simulink model "H2DFRL_LExCI_env"  (R2023a)
settings: Solver=FixedStepAuto  StartTime=0.0  StopTime=50  FixedStep=0.08  RelTol=1e-3
values from neighbouring files (symbols this model uses):
  action_mean_selector_ppo = 1:num_actions    [ReinforcementLearningBlockInit_H2DFRL.m]
  action_sampling_mode = 1    [ReinforcementLearningBlockInit_H2DFRL.m]
  action_selector_ddpg = 1:num_actions    [ReinforcementLearningBlockInit_H2DFRL.m]
  action_std_selector_ppo = 1:num_actions    [ReinforcementLearningBlockInit_H2DFRL.m]
  action_type = 1    [ReinforcementLearningBlockInit_H2DFRL.m]
  C2C_NMPC = init_C2C_NMPC_H2DF(C2C_NMPC.expdata)    [init_H2DFRL_GRU.m]
  LowerLimit = ([0.17e-3;350;-5;1e-3] - C2C_NMPC.Normalization.controls.mean)./(C2C_NMPC.Normalization.controls.std)    [init_H2DFRL_GRU.m]
  num_actions = 4    [ReinforcementLearningBlockInit_H2DFRL.m]
  rl_algorithm = 1    [ReinforcementLearningBlockInit_H2DFRL.m]
  UpperLimit = ([0.5e-3;900;2;5.5e-3] - C2C_NMPC.Normalization.controls.mean)./(C2C_NMPC.Normalization.controls.std)    [init_H2DFRL_GRU.m]
undefined symbols (not defined in the file or in its folder): CA50_offset, DiscIntNeverNeededParam, enable_CA50_noise, enable_CA50_offset, enable_IMEP_noise, enable_IMEP_offset, IMEP_offset, NUMBER_OF_ACTIONS
libraries: simulink x15, dspsrcs4 x4
(part 2 of 4)

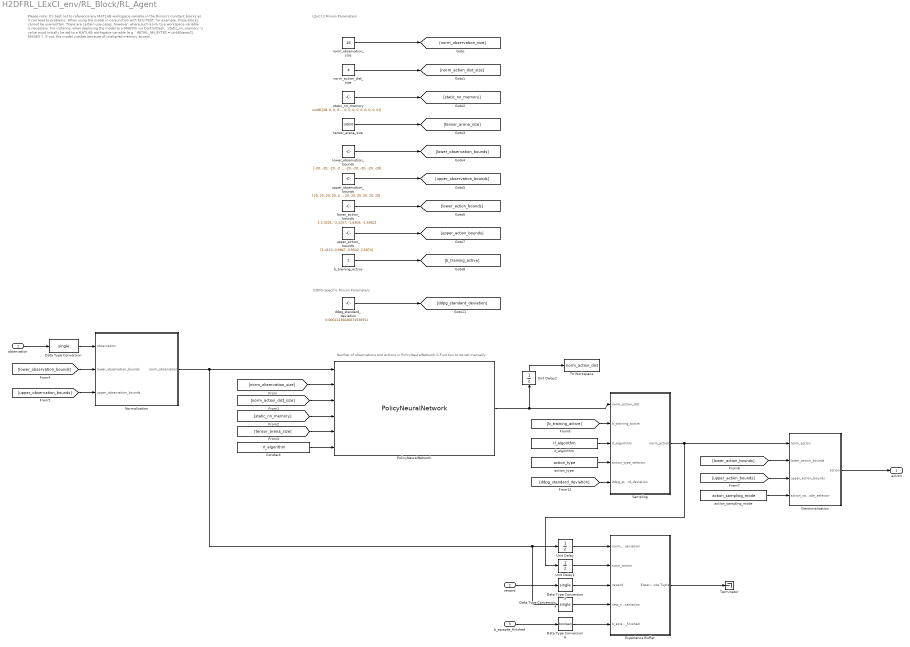
== system H2DFRL_LExCI_env/RL_Block/RL_Agent ==
  note: LExCI 2 Minion Parameters
  note: DDPG-Specific Minion Parameters
  note: Number of observations and actions in PolicyNeuralNetwork S-Function to be set manually.
  note: Please note:
      |
      | It's best not to reference any MATLAB workspace variable in the Minion's constant blocks as it can lead to
      | problems. When using the model in conjunction with ECU-TEST, for example, those blocks cannot be
      | overwritten.
      |
      | There are certain use-cases, however, where such a link to a workspace variable is necessary. For
      | instance, when deploying the model to a MABXIII via ControlDesk, `static_nn_memory`'s value must
      | initially be set to a MATLAB workspace variable (e.g. `INITIAL_NN_BYTES = uint8(zeros(1, 65536))`). If
      | not, the model crashes because of unaligned memory access.
  observation : Inport
  reward : Inport  Port=2
  b_episode_finished : Inport  Port=3
  Constant : Constant  Value=rl_algorithm  OutDataTypeStr=uint32
  Data Type Conversion : DataTypeConversion  OutDataTypeStr=single  SaturateOnIntegerOverflow=off  RndMeth=Floor
  Data Type Conversion3 : DataTypeConversion  OutDataTypeStr=single  SaturateOnIntegerOverflow=off  RndMeth=Floor
  Data Type Conversion4 : DataTypeConversion  OutDataTypeStr=single  SaturateOnIntegerOverflow=off  RndMeth=Floor
  Data Type Conversion6 : DataTypeConversion  OutDataTypeStr=boolean  SaturateOnIntegerOverflow=off  RndMeth=Floor
  Denormalization : Subsystem
  Experience Buffer : Subsystem
  Normalization : Subsystem
  PolicyNeuralNetwork : S-Function  InitFcn=try, set_param(gcb,'FunctionName','PolicyNeuralNetwork'), end  FunctionName=PolicyNeuralNetwork  SFunctionModules=PolicyNeuralNetwork_wrapper.cpp activations activations_common add add_common add_n arg_min_max assign_variable batch_to_space_nd broadcast_args broadcast_to call_once cast ceil circular_buffer circular_buffer_common comparisons concatenation conv conv_common cumsum depth_to_space depthwise_conv depthwise_conv_common dequantize dequantize_common detection_postprocess div elementwise elu ethosu exp expand_dims fill floor floor_div floor_mod fully_connected fully_connected_common gather gather_nd hard_swish hard_swish_common if kernel_runner kernel_util_micro l2norm l2_pool_2d leaky_relu leaky_relu_common logical logical_common logistic logistic_common log_softmax lstm_eval maximum_minimum micro_tensor_utils mirror_pad mul mul_common neg pack pad pooling pooling_common prelu prelu_common quantize quantize_common read_variable reduce reduce_common reshape resize_bilinear resize_nearest_neighbor round shape slice softmax softmax_common space_to_batch_nd space_to_depth split split_v squared_difference squeeze strided_slice sub sub_common svdf svdf_common tanh transpose transpose_conv unidirectional_sequence_lstm unpack var_handle while zeros_like flatbuffer_conversions op_resolver tensor_utils error_reporter schema_utils kernel_util portable_tensor_utils quantization_util common memory_helpers all_ops_resolver micro_graph micro_error_reporter micro_context micro_profiler test_helpers recording_micro_allocator micro_interpreter micro_time micro_resource_variable test_helper_custom_ops flatbuffer_utils mock_micro_graph debug_log micro_allocation_info system_setup micro_allocator micro_string micro_utils fake_micro_context persistent_arena_buffer_allocator recording_single_arena_buffer_allocator non_persistent_arena_buffer_allocator single_arena_buffer_allocator greedy_memory_planner linear_memory_planner non_persistent_buffer_planner_shim  SFunctionDeploymentMode=off  EnableBusSupport=off  mask(S-Function Builder){}
      mask help: Simulink:masks:SFunctionBuilder_MD
      mask init:
      | val = [[.9  0.75 0.75 1 1 .9 .9 1]',[1 1 0.75 0.75 .9 .9 1 .9]'];try , sys = get_param(gcb,'SfunBuilderFcnName');if isempty(sys), sys = get_param(gcb,'FunctionName'); end,catch, sys = get_param(gcb,'FunctionName'); end
      settings: CopyFcn=set_param(gcbh,'LinkStatus','none')  PreSaveFcn=try, set_param(gcb,'FunctionName','PolicyNeuralNetwork'), end  OpenFcn=sfunctionwizard(gcbh)
      mask Display: plot(val(:,1),val(:,2)),disp(sys),port_label('input',1,'norm_observation'),port_label('input',2,'norm_observation_size'),port_label('input',3,'norm_action_dist_size'),port_label('input',4,'static_nn_memory'),port_label('input',5,'tensor_arena_size'),port_label('input',6,'rl_algorithm'),port_label('output',1,'norm_action_dist')
  Sampling : Subsystem
  Terminator : Terminator
  To Workspace : ToWorkspace  VariableName=norm_action_dist  SampleTime=-1
  Unit Delay : UnitDelay  InitialCondition=-1*ones(16,1)  SampleTime=-1  HasFrameUpgradeWarning=on
  Unit Delay1 : UnitDelay  InitialCondition=-1*ones(4,1)  SampleTime=-1  HasFrameUpgradeWarning=on
  Unit Delay2 : UnitDelay  InitialCondition=-1*ones(4,1)  SampleTime=-1  HasFrameUpgradeWarning=on
  action_sampling_mode : Constant  Value=action_sampling_mode  OutDataTypeStr=uint8
  action_type : Constant  Value=action_type  OutDataTypeStr=uint8
  b_training_active : Constant  OutDataTypeStr=boolean
  ddpg_standard_deviation : Constant  Value=0.00011236636674536911  OutDataTypeStr=single
  lower_action_bounds : Constant  Value=[-2.3201, -2.1257, -1.8309, -1.6562]  OutDataTypeStr=single
  lower_observation_bounds : Constant  Value=[-20, -20, -20, -20, -20, -20, -20, -20, -20, -20, -20, -20, -20, -20, -20, -20]  OutDataTypeStr=single
  norm_action_dist_size : Constant  Value=4  OutDataTypeStr=uint32
  norm_observation_size : Constant  Value=16  OutDataTypeStr=uint32
  rl_algorithm : Constant  Value=rl_algorithm  OutDataTypeStr=uint8
  static_nn_memory : Constant  Value=uint8([28, 0, 0, 0, 84, 70, 76, 51, 0, 0, 18, 0, 28, 0, 24, 0, 20, 0, 16, 0, 12, 0, 8, 0, 0, 0, 4, 0, 18, 0, 0, 0, 24, 0, 0, 0, 104, 0, 0, 0, 140, 87, 0, 0, 156, 87, 0, 0, 228, 91, 0, 0, 3, 0, 0, 0, 2, 0, 0, 0, 44, 0, 0, 0, 4, 0, 0, 0, 40, 167, 255, 255, 12, 0, 0, 0, 4, 0, 0, 0, 19, 0, 0, 0, 67, 79, 78, 86, 69, 82, 83, 73, 79, 78, 95, 77, 69, 84, 65, 68, 65, 84, 65, 0, 76, 167, 255, 255, 11, 0, 0, 0, 4, 0, 0, 0, 19, 0, 0, 0, 109, 105, 110, 95, 114, 117, 110, 116, 105, 109, 101, 95, 118, 101, 114, 115, 105, 111, 110, 0, 13, 0, 0, 0, 32, 87, 0, 0, 0, 87, 0, 0, 232, 82, 0, 0, 216, 81, 0, 0, 200, 17, 0, 0, 184, 16, 0, 0, 168, 0, 0, 0, 160, 0, 0, 0, 152, 0, 0, 0, 144, 0, 0, 0, 136, 0, 0, 0, 104, 0, 0, 0, 4, 0, 0, 0, 54, 169, 255, 255, 4, 0, 0, 0, 84, 0, 0, 0, 12, 0, 0, 0, 8, 0, 14, 0, 8, 0, 4, 0, 8, 0, 0, 0, 16, 0, 0, 0, 36, 0, 0, 0, 0, 0, 6, 0, 8, 0, 4, 0, 6, 0, 0, 0, 4, 0, 0, 0, 0, 0, 0, 0, 0, 0, 10, 0, 16, 0, 12, 0, 8, 0, 4, 0, 10, 0, 0, 0, 2, 0, 0, 0, 2, 0, 0, 0, 4, 0, 0, 0, 6, 0, 0, 0, 50, 46, 49, 49, 46, 48, 0, 0, 150, 169, 255, 255, 4, 0, 0, 0, 16, 0, 0, 0, 49, 46, 53, 46, 48, 0, 0, 0, 0, 0, 0, 0, 0, 0, 0, 0, 80, 165, 255, 255, 84, 165, 255, 255, 88, 165, 255, 255, 92, 165, 255, 255, 194, 169, 255, 255, 4, 0, 0, 0, 0, 16, 0, 0, 209, 12, 15, 63, 107, 121, 33, 63, 92, 40, 22, 191, 85, 158, 60, 63, 75, 14, 66, 61, 94, 22, 151, 60, 63, 159, 19, 63, 41, 61, 196, 190, 78, 51, 178, 190, 40, 117, 157, 62, 38, 27, 46, 63, 129, 239, 240, 190, 20, 116, 244, 62, 126, 176, 40, 63, 56, 160, 7, 191, 196, 106, 28, 191, 145, 7, 172, 155, 50, 94, 17, 30, 228, 111, 15, 35, 218, 1, 32, 157, 131, 165, 85, 170, 236, 130, 207, 172, 207, 18, 135, 184, 100, 3, 163, 166, 80, 110, 11, 22, 102, 215, 86, 143, 126, 110, 70, 27, 224, 187, 57, 33, 150, 18, 111, 159, 203, 114, 13, 155, 42, 41, 242, 151, 222, 13, 5, 20, 40, 179, 141, 62, 78, 24, 190, 62, 167, 182, 179, 190, 191, 185, 79, 61, 115, 107, 177, 190, 190, 66, 165, 190, 246, 192, 251, 62, 132, 114, 8, 191, 191, 223, 202, 189, 117, 213, 199, 62, 235, 76, 196, 62, 10, 235, 153, 190, 134, 127, 5, 62, 100, 124, 5, 63, 184, 228, 109, 190, 107, 218, 135, 190, 78, 215, 85, 15, 105, 50, 86, 15, 85, 26, 86, 143, 98, 136, 86, 143, 95, 243, 86, 15, 52, 234, 85, 15, 217, 24, 87, 143, 33, 159, 87, 143, 128, 84, 86, 15, 93, 204, 85, 15, 62, 78, 87, 143, 161, 17, 86, 143, 0, 107, 85, 143, 194, 106, 86, 143, 228, 69, 86, 143, 216, 92, 85, 15, 206, 236, 29, 63, 218, 110, 202, 62, 247, 13, 20, 191, 185, 38, 150, 62, 88, 151, 135, 190, 71, 141, 165, 190, 154, 54, 87, 63, 154, 137, 5, 191, 250, 73, 200, 190, 2, 242, 136, 62, 197, 176, 36, 63, 59, 22, 10, 191, 61, 122, 4, 63, 65, 199, 21, 63, 72, 5, 210, 190, 171, 13, 4, 191, 253, 241, 16, 63, 241, 172, 197, 62, 102, 78, 150, 190, 26, 38, 254, 61, 113, 87, 202, 190, 41, 100, 233, 190, 78, 233, 4, 63, 102, 124, 68, 191, 189, 170, 185, 190, 209, 39, 95, 62, 129, 40, 50, 63, 191, 167, 79, 190, 187, 180, 78, 62, 29, 233, 46, 63, 203, 162, 179, 190, 39, 147, 234, 190, 89, 219, 17, 63, 202, 65, 247, 62, 140, 34, 152, 190, 138, 188, 6, 63, 18, 149, 8, 190, 33, 169, 115, 190, 113, 88, 59, 63, 46, 250, 64, 191, 0, 81, 44, 190, 35, 213, 134, 62, 99, 240, 233, 62, 1, 90, 147, 190, 73, 35, 198, 62, 11, 239, 239, 62, 177, 67, 161, 190, 246, 227, 194, 190, 190, 87, 9, 63, 183, 239, 42, 63, 36, 230, 241, 190, 111, 131, 248, 62, 114, 46, 98, 60, 81, 255, 24, 62, 35, 109, 18, 63, 204, 79, 92, 190, 252, 91, 137, 190, 39, 128, 175, 62, 118, 198, 58, 63, 22, 31, 247, 190, 160, 243, 1, 63, 55, 81, 4, 63, 70, 78, 11, 191, 6, 89, 27, 191, 209, 69, 86, 15, 187, 73, 86, 15, 200, 158, 85, 15, 238, 214, 85, 15, 142, 49, 86, 15, 62, 39, 86, 143, 85, 24, 86, 143, 62, 191, 85, 143, 66, 129, 85, 15, 211, 66, 86, 143, 18, 228, 85, 143, 194, 110, 85, 15, 238, 183, 86, 15, 91, 129, 87, 15, 247, 74, 86, 143, 217, 44, 87, 15, 9, 154, 83, 62, 212, 111, 254, 62, 11, 173, 8, 191, 215, 232, 101, 62, 160, 169, 31, 190, 69, 126, 101, 61, 219, 255, 105, 63, 235, 75, 17, 191, 188, 227, 147, 190, 95, 57, 152, 62, 13, ...(+225968 chars)])  OutDataTypeStr=uint8
  tensor_arena_size : Constant  Value=100000  OutDataTypeStr=uint32
  upper_action_bounds : Constant  Value=[1.4113, 0.9867, 0.9542, 2.1874]  OutDataTypeStr=single
  upper_observation_bounds : Constant  Value=[20, 20, 20, 20, 20, 20, 20, 20, 20, 20, 20, 20, 20, 20, 20, 20]  OutDataTypeStr=single
  action : Outport
  wires:
  upper_action_bounds/1 -> [upper_action_bounds]
  PolicyNeuralNetwork/1 -> Unit Delay2/1, Sampling/1(norm_action_dist)
  upper_observation_bounds/1 -> [upper_observation_bounds]
  lower_action_bounds/1 -> [lower_action_bounds]
  [upper_observation_bounds] -> Normalization/3(upper_observation_bounds)
  [tensor_arena_size] -> PolicyNeuralNetwork/5
  b_episode_finished/1 -> Data Type Conversion6/1
  Unit Delay/1 -> Experience Buffer/1(norm_observation)
  [norm_observation_size] -> PolicyNeuralNetwork/2
  Data Type Conversion6/1 -> Experience Buffer/5(b_episode_finished)
  Unit Delay1/1 -> Experience Buffer/2(norm_action)
  Data Type Conversion3/1 -> Experience Buffer/3(reward)
  norm_observation_size/1 -> [norm_observation_size]
  Data Type Conversion/1 -> Normalization/1(observation)
  lower_observation_bounds/1 -> [lower_observation_bounds]
  Data Type Conversion4/1 -> Experience Buffer/4(new_norm_observation)
  reward/1 -> Data Type Conversion3/1
  norm_action_dist_size/1 -> [norm_action_dist_size]
  static_nn_memory/1 -> [static_nn_memory]
  Normalization/1(norm_observation) -> Unit Delay/1, Data Type Conversion4/1, PolicyNeuralNetwork/1
  observation/1 -> Data Type Conversion/1
  [norm_action_dist_size] -> PolicyNeuralNetwork/3
  [lower_observation_bounds] -> Normalization/2(lower_observation_bounds)
  tensor_arena_size/1 -> [tensor_arena_size]
  Experience Buffer/1(Experience Tuple) -> Terminator/1
  Sampling/1(norm_action) -> Unit Delay1/1, Denormalization/1(norm_action)
  Denormalization/1(action) -> action/1
  [lower_action_bounds] -> Denormalization/2(lower_action_bounds)
  [upper_action_bounds] -> Denormalization/3(upper_action_bounds)
  [static_nn_memory] -> PolicyNeuralNetwork/4
  b_training_active/1 -> [b_training_active]
  [b_training_active] -> Sampling/2(b_training_active)
  ddpg_standard_deviation/1 -> [ddpg_standard_deviation]
  action_sampling_mode/1 -> Denormalization/4(action_sampling_mode_selector)
  action_type/1 -> Sampling/4(action_type_selector)
  rl_algorithm/1 -> Sampling/3(rl_algorithm)
  [ddpg_standard_deviation] -> Sampling/5(ddpg_standard_deviation)
  Constant/1 -> PolicyNeuralNetwork/6
  Unit Delay2/1 -> To Workspace/1
